simulink library "sf_atomic_sensor_lib"  (R2017b)
settings: Solver=ode45  StartTime=0.0  StopTime=10.0  RelTol=1e-3  EnableMultiTasking=on
undefined symbols (not defined in the file): HIGH, LOW
settings Model: Creator=The MathWorks, Inc.  LastModifiedBy=The MathWorks, Inc.
settings DataIOCC: LimitDataPoints=on  SaveFormat=Array  SignalLoggingSaveFormat=ModelDataLogs
settings OptimizationCC: ExpressionDepthLimit=2147483647  LifeSpan=inf
settings DebuggingCC: UnderspecifiedInitializationDetection=Classic  MergeDetectMultiDrivingBlocksExec=none  SolverPrmCheckMsg=warning  FcnCallInpInsideContextMsg=warning  StateNameClashWarn=warning  SFUnexpectedBacktrackingDiag=warning  SFNoUnconditionalDefaultTransitionDiag=warning  SFExecutionAtInitializationDiag=none
settings HardwareCC: ProdBitPerPointer=32  ProdBitPerSizeT=32  ProdBitPerPtrDiffT=32  ProdLargestAtomicFloat=None  ProdIntDivRoundTo=Undefined  ProdEndianess=Unspecified  ProdWordSize=32  ProdHWDeviceType=32-bit Generic
settings ModelReferenceCC: PropagateSignalLabelsOutOfModel=off
settings CodeAppCC: StateflowObjectComments=on
settings GRTTargetCC: TargetLangStandard=C89/C90 (ANSI)  GeneratePreprocessorConditionals=Disable all  CombineOutputUpdateFcns=off  GRTInterface=on
settings ConfigComp: CovMetricSettings=dw  CovHtmlReporting=on  CovSaveCumulativeToWorkspaceVar=on  CovSaveSingleToWorkspaceVar=on  CovExternalEMLEnable=off

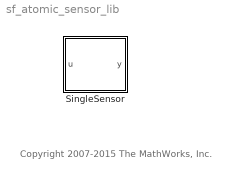
== system sf_atomic_sensor_lib ==
  note: Copyright 2007-2015 The MathWorks, Inc.
  SingleSensor : Stateflow chart  TreatAsAtomicUnit=on

== stateflow chart sf_atomic_sensor_lib/SingleSensor ==
  state Fail
    en, du: y = 0;
  state OK
    en, du: y = u;
  state FailOnce
  state yn = readingOK [function]
    (default) -> (junction 19) : {yn = (u > LOW && u < HIGH);}
  state yn = inFailed [function]
    (default) -> (junction 23) : {yn = in(Fail);}
  (default) -> OK
  OK -> FailOnce : [!readingOK()]
  FailOnce -> Fail [order 1] : [after(1,sec)]
  FailOnce -> OK [order 2] : [readingOK()]
  data: yn function_output double; yn function_output double; u input; y output double; HIGH parameter; LOW parameter
